simulink model "model_vec"  (R2022b)
settings: Solver=ode4  StartTime=0.0  StopTime=1.3  FixedStep=10e-6  RelTol=1e-3
InitFcn:
  | model_
values from neighbouring files (symbols this model uses):
  f = 50    [model_.m]
  i1dn = psi2n/Lm    [model_.m]
  i1qn = sqrt(Inmax^2-i1dn^2)    [model_.m]
  J = 0.4    [model_.m]
  L1 = L1sigma+Lm    (= 0.08477)    [model_.m]
  L1sigma = 2.27e-3    (= 0.00227)    [model_.m]
  L2 = L2sigma+Lm    (= 0.08477)    [model_.m]
  L2sigma = 2.27e-3    (= 0.00227)    [model_.m]
  Lm = 82.5e-3    (= 0.0825)    [model_.m]
  pp = 2    [model_.m]
  psi2n = sqrt(psi2nre^2+psi2nim^2)    [model_.m]
  R1 = 370e-3    (= 0.37)    [model_.m]
  R2 = 225e-3    (= 0.225)    [model_.m]
  R2_vec_model = 225e-3    (= 0.225)    [model_.m]
  sigma = 1-Lm^(2)/(L1*L2)    (= 0.0528396032209)    [model_.m]
  svmFrequency = 10000    [model_.m]
  Us = 400    [model_.m]
libraries: eeTransforms x16, spsMeanLib x7, slpidlib x4, simulink x2, dspsigops x2
(part 3 of 3)

== system model_vec/ASM1/i2 ==
  psi_2alpha : Inport
  psi_2beta : Inport  Port=2
  i_1_alpha_beta : Inport  Port=3
  Add2 : Sum  Inputs=+-
  Constant6 : Constant  Value=Lm
  Constant7 : Constant  Value=L2
  Divide4 : Product  Inputs=**
  Divide5 : Product  Inputs=*/
  Mux2 : Mux  Inputs=2
  i_2alpha_beta : Outport
  wires:
  i_1_alpha_beta/1 -> Divide4/1
  Divide5/1 -> i_2alpha_beta/1
  Constant7/1 -> Divide5/2
  psi_2beta/1 -> Mux2/2
  Divide4/1 -> Add2/2
  Constant6/1 -> Divide4/2
  Add2/1 -> Divide5/1
  Mux2/1 -> Add2/1
  psi_2alpha/1 -> Mux2/1

== system model_vec/ASM2/ClarkeTransform1 ==
  u_1source : Inport
  K : Inport  Port=2
  Add1 : Sum  Inputs=+++
  Add2 : Sum  Inputs=+++
  Demux4 : Demux  Outputs=3
  Demux5 : Demux  Outputs=3
  Divide2 : Product  Inputs=**
  Divide3 : Product  Inputs=**
  Gain : Gain  Gain=-1/2
  Gain1 : Gain  Gain=-1/2
  Gain2 : Gain  Gain=-sqrt(3)/2
  Gain3 : Gain  Gain=sqrt(3)/2
  Gain4 : Gain
  Gain5 : Gain  Gain=0
  Mux2 : Mux  Inputs=2
  u1_in_alpha_beta : Outport
  wires:
  Demux4/1 -> Gain4/1  "ua"
  Divide2/1 -> Mux2/1  "u_1alpha"
  [K_ClarkeTransform] -> Divide2/2
  Add1/1 -> Divide2/1
  Demux4/2 -> Gain/1  "ub"
  Divide3/1 -> Mux2/2  "u_1beta"
  Gain5/1 -> Add2/1
  Gain/1 -> Add1/2
  Demux5/1 -> Gain5/1  "ua"
  Gain3/1 -> Add2/3
  [K_ClarkeTransform] -> Divide3/2
  Gain2/1 -> Add2/2
  Gain1/1 -> Add1/3
  Demux5/2 -> Gain2/1  "ub"
  Demux5/3 -> Gain3/1  "uc"
  Add2/1 -> Divide3/1
  Gain4/1 -> Add1/1
  u_1source/1 -> Demux5/1, Demux4/1
  K/1 -> [K_ClarkeTransform]
  Mux2/1 -> u1_in_alpha_beta/1
  Demux4/3 -> Gain1/1  "uc"

== system model_vec/ASM2/Mh ==
  i_1alpha : Inport
  i_1beta : Inport  Port=2
  phi_2alpha : Inport  Port=3
  phi_2beta : Inport  Port=4
  Add : Sum  Inputs=+-
  Constant : Constant  Value=3/2
  Constant1 : Constant  Value=pp
  Constant2 : Constant  Value=Lm
  Constant3 : Constant  Value=L2
  Divide{,1,3..5} (5 alike) : Product  Inputs=**
  Divide2 : Product  Inputs=*/
  Mh : Outport
  wires:
  Constant/1 -> Divide/1
  Constant1/1 -> Divide/2
  Divide/1 -> Divide1/1
  Constant2/1 -> Divide2/1
  Constant3/1 -> Divide2/2
  Divide2/1 -> Divide1/2
  Divide1/1 -> Divide3/2
  phi_2alpha/1 -> Divide4/2
  i_1beta/1 -> Divide4/1
  Divide4/1 -> Add/1
  phi_2beta/1 -> Divide5/1
  i_1alpha/1 -> Divide5/2
  Divide5/1 -> Add/2
  Add/1 -> Divide3/1
  Divide3/1 -> Mh/1

== system model_vec/ASM2/Mh Static ==
  Slip : Inport
  Add3 : Sum
  Add4 : Sum
  Add6 : Sum
  Constant10 : Constant  Value=230^(2)
  Constant11 : Constant  Value=pp
  Constant14 : Constant  Value=2*pi*f
  Constant15 : Constant  Value=R1
  Constant16 : Constant  Value=R2
  Constant21 : Constant  Value=2*pi*f
  Constant22 : Constant  Value=L1sigma
  Constant23 : Constant  Value=L2sigma
  Constant8 : Constant  Value=3
  Constant9 : Constant  Value=R2
  Divide10 : Product  Inputs=/*
  Divide11 : Product  Inputs=*/
  Divide15 : Product  Inputs=**
  Divide6 : Product  Inputs=****
  Divide7 : Product  Inputs=*/
  Divide8 : Product  Inputs=**
  Math Function : Math  Operator=square
  Math Function2 : Math  Operator=square
  Reprezentace s s*omega1*L2sigma : Subsystem
  Mh Static : Outport
  wires:
  Slip/1 -> Divide8/2, Divide11/2
  Constant11/1 -> Divide6/4
  Constant10/1 -> Divide6/3
  Add4/1 -> Math Function/1
  Constant16/1 -> Divide11/1
  Constant9/1 -> Divide6/2
  Constant23/1 -> Add6/2
  Constant15/1 -> Add4/1
  Divide15/1 -> Math Function2/1
  Divide8/1 -> Divide7/2
  Constant14/1 -> Divide8/1
  Math Function/1 -> Add3/1
  Divide7/1 -> Divide10/2
  Divide10/1 -> Mh Static/1
  Divide11/1 -> Add4/2
  Constant22/1 -> Add6/1
  Add6/1 -> Divide15/1
  Constant8/1 -> Divide6/1
  Constant21/1 -> Divide15/2
  Add3/1 -> Divide10/1
  Divide6/1 -> Divide7/1
  Math Function2/1 -> Add3/2

== system model_vec/ASM2/Slip ==
  omega : Inport
  Add2 : Sum  Inputs=+-
  Constant12 : Constant  Value=2*pi*f
  Constant13 : Constant  Value=2*pi*f
  Divide9 : Product  Inputs=*/
  Slip : Outport
  wires:
  omega/1 -> Add2/2  "Omega"
  Divide9/1 -> Slip/1
  Constant12/1 -> Add2/1
  Add2/1 -> Divide9/1
  Constant13/1 -> Divide9/2

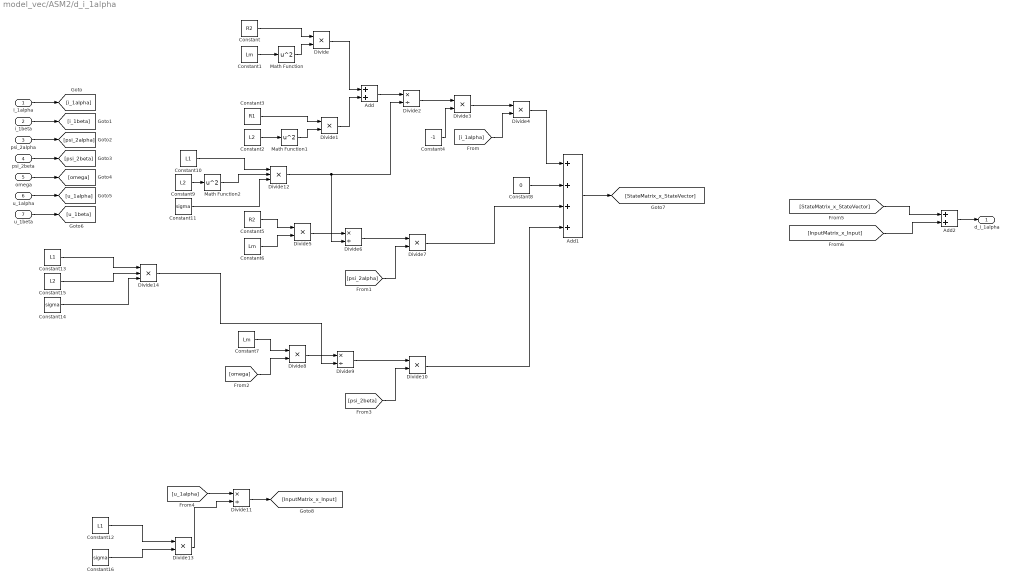
== system model_vec/ASM2/d_i_1alpha ==
  i_1alpha : Inport
  i_1beta : Inport  Port=2
  psi_2alpha : Inport  Port=3
  psi_2beta : Inport  Port=4
  omega : Inport  Port=5
  u_1alpha : Inport  Port=6
  u_1beta : Inport  Port=7
  Add : Sum
  Add1 : Sum  Inputs=++++
  Add2 : Sum
  Constant : Constant  Value=R2
  Constant1 : Constant  Value=Lm
  Constant10 : Constant  Value=L1
  Constant11 : Constant  Value=sigma
  Constant12 : Constant  Value=L1
  Constant13 : Constant  Value=L1
  Constant14 : Constant  Value=sigma
  Constant15 : Constant  Value=L2
  Constant16 : Constant  Value=sigma
  Constant2 : Constant  Value=L2
  Constant3 : Constant  Value=R1
  Constant4 : Constant  Value=-1
  Constant5 : Constant  Value=R2
  Constant6 : Constant  Value=Lm
  Constant7 : Constant  Value=Lm
  Constant8 : Constant  Value=0
  Constant9 : Constant  Value=L2
  Divide{,1,3..5,7..8,10,13} (9 alike) : Product  Inputs=**
  Divide{2,6,9,11} (4 alike) : Product  Inputs=*/
  Divide12 : Product  Inputs=***
  Divide14 : Product  Inputs=***
  Math Function : Math  Operator=square
  Math Function1 : Math  Operator=square
  Math Function2 : Math  Operator=square
  d_i_1alpha : Outport
  wires:
  Constant1/1 -> Math Function/1
  Constant/1 -> Divide/1
  Math Function/1 -> Divide/2
  Divide/1 -> Add/1
  Constant2/1 -> Math Function1/1
  Constant3/1 -> Divide1/1
  Math Function1/1 -> Divide1/2
  Divide1/1 -> Add/2
  Add/1 -> Divide2/1
  Constant4/1 -> Divide3/2
  Divide2/1 -> Divide3/1
  Divide3/1 -> Divide4/1
  i_1alpha/1 -> [i_1alpha]
  i_1beta/1 -> [i_1beta]
  psi_2alpha/1 -> [psi_2alpha]
  psi_2beta/1 -> [psi_2beta]
  omega/1 -> [omega]
  [i_1alpha] -> Divide4/2
  Divide4/1 -> Add1/1
  Constant5/1 -> Divide5/1
  Constant6/1 -> Divide5/2
  Divide5/1 -> Divide6/1
  Divide6/1 -> Divide7/1
  [psi_2alpha] -> Divide7/2
  Divide7/1 -> Add1/3
  Constant7/1 -> Divide8/1
  [omega] -> Divide8/2
  Divide8/1 -> Divide9/1
  Divide9/1 -> Divide10/1
  [psi_2beta] -> Divide10/2
  Divide10/1 -> Add1/4
  Constant8/1 -> Add1/2
  u_1alpha/1 -> [u_1alpha]
  u_1beta/1 -> [u_1beta]
  Add1/1 -> [StateMatrix_x_StateVector]
  [u_1alpha] -> Divide11/1
  Divide11/1 -> [InputMatrix_x_Input]
  [StateMatrix_x_StateVector] -> Add2/1
  [InputMatrix_x_Input] -> Add2/2
  Add2/1 -> d_i_1alpha/1
  Constant9/1 -> Math Function2/1
  Constant10/1 -> Divide12/1
  Math Function2/1 -> Divide12/2
  Constant11/1 -> Divide12/3
  Divide12/1 -> Divide6/2, Divide2/2
  Constant14/1 -> Divide14/3
  Constant13/1 -> Divide14/1
  Constant15/1 -> Divide14/2
  Constant12/1 -> Divide13/1
  Constant16/1 -> Divide13/2
  Divide13/1 -> Divide11/2
  Divide14/1 -> Divide9/2

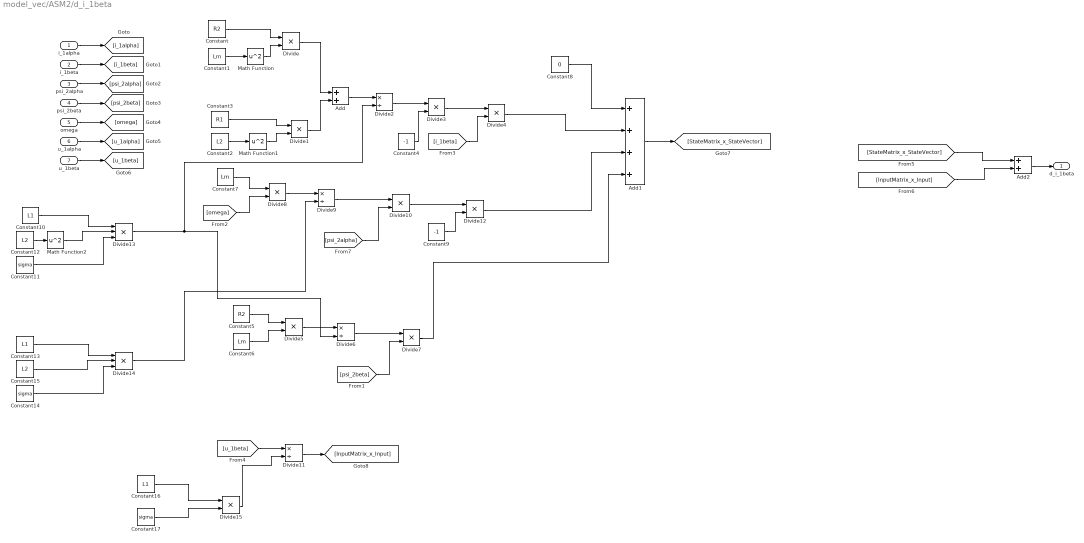
== system model_vec/ASM2/d_i_1beta ==
  i_1alpha : Inport
  i_1beta : Inport  Port=2
  psi_2alpha : Inport  Port=3
  psi_2beta : Inport  Port=4
  omega : Inport  Port=5
  u_1alpha : Inport  Port=6
  u_1beta : Inport  Port=7
  Add : Sum
  Add1 : Sum  Inputs=++++
  Add2 : Sum
  Constant : Constant  Value=R2
  Constant1 : Constant  Value=Lm
  Constant10 : Constant  Value=L1
  Constant11 : Constant  Value=sigma
  Constant12 : Constant  Value=L2
  Constant13 : Constant  Value=L1
  Constant14 : Constant  Value=sigma
  Constant15 : Constant  Value=L2
  Constant16 : Constant  Value=L1
  Constant17 : Constant  Value=sigma
  Constant2 : Constant  Value=L2
  Constant3 : Constant  Value=R1
  Constant4 : Constant  Value=-1
  Constant5 : Constant  Value=R2
  Constant6 : Constant  Value=Lm
  Constant7 : Constant  Value=Lm
  Constant8 : Constant  Value=0
  Constant9 : Constant  Value=-1
  Divide{,1,3..5,7..8,10,12,15} (10 alike) : Product  Inputs=**
  Divide{2,6,9,11} (4 alike) : Product  Inputs=*/
  Divide13 : Product  Inputs=***
  Divide14 : Product  Inputs=***
  Math Function : Math  Operator=square
  Math Function1 : Math  Operator=square
  Math Function2 : Math  Operator=square
  d_i_1beta : Outport
  wires:
  Add2/1 -> d_i_1beta/1
  [InputMatrix_x_Input] -> Add2/2
  [StateMatrix_x_StateVector] -> Add2/1
  Divide11/1 -> [InputMatrix_x_Input]
  [u_1beta] -> Divide11/1
  Add1/1 -> [StateMatrix_x_StateVector]
  u_1beta/1 -> [u_1beta]
  u_1alpha/1 -> [u_1alpha]
  Constant8/1 -> Add1/1
  Divide10/1 -> Divide12/1
  [psi_2alpha] -> Divide10/2
  Divide9/1 -> Divide10/1
  Divide8/1 -> Divide9/1
  [omega] -> Divide8/2
  Constant7/1 -> Divide8/1
  Divide7/1 -> Add1/4
  [psi_2beta] -> Divide7/2
  Divide6/1 -> Divide7/1
  Divide5/1 -> Divide6/1
  Constant6/1 -> Divide5/2
  Constant5/1 -> Divide5/1
  Divide4/1 -> Add1/2
  [i_1beta] -> Divide4/2
  omega/1 -> [omega]
  psi_2beta/1 -> [psi_2beta]
  psi_2alpha/1 -> [psi_2alpha]
  i_1beta/1 -> [i_1beta]
  i_1alpha/1 -> [i_1alpha]
  Divide3/1 -> Divide4/1
  Divide2/1 -> Divide3/1
  Constant4/1 -> Divide3/2
  Add/1 -> Divide2/1
  Divide1/1 -> Add/2
  Math Function1/1 -> Divide1/2
  Constant3/1 -> Divide1/1
  Constant2/1 -> Math Function1/1
  Divide/1 -> Add/1
  Math Function/1 -> Divide/2
  Constant/1 -> Divide/1
  Constant1/1 -> Math Function/1
  Constant9/1 -> Divide12/2
  Divide12/1 -> Add1/3
  Constant10/1 -> Divide13/1
  Constant11/1 -> Divide13/3
  Math Function2/1 -> Divide13/2
  Divide13/1 -> Divide6/2, Divide2/2
  Constant12/1 -> Math Function2/1
  Divide14/1 -> Divide9/2
  Constant14/1 -> Divide14/3
  Constant15/1 -> Divide14/2
  Constant13/1 -> Divide14/1
  Constant16/1 -> Divide15/1
  Divide15/1 -> Divide11/2
  Constant17/1 -> Divide15/2

== system model_vec/ASM2/d_psi_2alpha ==
  note: je to jen pro úplnost
  i_1alpha : Inport
  i_1beta : Inport  Port=2
  psi_2alpha : Inport  Port=3
  psi_2beta : Inport  Port=4
  omega : Inport  Port=5
  u_1alpha : Inport  Port=6
  u_1beta : Inport  Port=7
  Add1 : Sum  Inputs=++++
  Add2 : Sum
  Constant : Constant  Value=0
  Constant1 : Constant  Value=-1
  Constant2 : Constant  Value=-1
  Constant3 : Constant  Value=R2
  Constant4 : Constant  Value=L2
  Constant5 : Constant  Value=Lm
  Constant6 : Constant  Value=R2
  Constant7 : Constant  Value=L2
  Constant8 : Constant  Value=0
  Divide{,1,3..5,7} (6 alike) : Product  Inputs=**
  Divide2 : Product  Inputs=*/
  Divide6 : Product  Inputs=*/
  d_psi_2alpha : Outport
  wires:
  i_1alpha/1 -> [i_1alpha]
  i_1beta/1 -> [i_1beta]
  psi_2alpha/1 -> [psi_2alpha]
  psi_2beta/1 -> [psi_2beta]
  omega/1 -> [omega]
  Constant8/1 -> Add1/2
  u_1alpha/1 -> [u_1alpha]
  u_1beta/1 -> [u_1beta]
  Add1/1 -> [StateMatrix_x_StateVector]
  Constant/1 -> [InputMatrix_x_Input]
  [StateMatrix_x_StateVector] -> Add2/1
  [InputMatrix_x_Input] -> Add2/2
  Add2/1 -> d_psi_2alpha/1
  [omega] -> Divide/1
  Constant1/1 -> Divide/2
  Divide/1 -> Divide1/1
  [psi_2beta] -> Divide1/2
  Divide1/1 -> Add1/4
  Constant2/1 -> Divide3/2
  Divide2/1 -> Divide3/1
  Constant3/1 -> Divide2/1
  Constant4/1 -> Divide2/2
  Divide3/1 -> Divide4/1
  [psi_2alpha] -> Divide4/2
  Divide4/1 -> Add1/3
  Divide5/1 -> Divide6/1
  Constant5/1 -> Divide5/1
  Constant6/1 -> Divide5/2
  Constant7/1 -> Divide6/2
  Divide6/1 -> Divide7/1
  [i_1alpha] -> Divide7/2
  Divide7/1 -> Add1/1

== system model_vec/ASM2/d_psi_2beta ==
  i_1alpha : Inport
  i_1beta : Inport  Port=2
  psi_2alpha : Inport  Port=3
  psi_2beta : Inport  Port=4
  omega : Inport  Port=5
  u_1alpha : Inport  Port=6
  u_1beta : Inport  Port=7
  Add1 : Sum  Inputs=++++
  Add2 : Sum
  Constant : Constant  Value=0
  Constant2 : Constant  Value=-1
  Constant3 : Constant  Value=R2
  Constant4 : Constant  Value=L2
  Constant5 : Constant  Value=Lm
  Constant6 : Constant  Value=R2
  Constant7 : Constant  Value=L2
  Constant8 : Constant  Value=0
  Divide{1,3..5,7} (5 alike) : Product  Inputs=**
  Divide2 : Product  Inputs=*/
  Divide6 : Product  Inputs=*/
  d_psi_2beta : Outport
  wires:
  Divide7/1 -> Add1/2
  [i_1beta] -> Divide7/2
  Divide6/1 -> Divide7/1
  Constant7/1 -> Divide6/2
  Constant6/1 -> Divide5/2
  Constant5/1 -> Divide5/1
  Divide5/1 -> Divide6/1
  Divide4/1 -> Add1/4
  [psi_2beta] -> Divide4/2
  Divide3/1 -> Divide4/1
  Constant4/1 -> Divide2/2
  Constant3/1 -> Divide2/1
  Divide2/1 -> Divide3/1
  Constant2/1 -> Divide3/2
  Divide1/1 -> Add1/3
  [psi_2alpha] -> Divide1/2
  Add2/1 -> d_psi_2beta/1
  [InputMatrix_x_Input] -> Add2/2
  [StateMatrix_x_StateVector] -> Add2/1
  Constant/1 -> [InputMatrix_x_Input]
  Add1/1 -> [StateMatrix_x_StateVector]
  u_1beta/1 -> [u_1beta]
  u_1alpha/1 -> [u_1alpha]
  Constant8/1 -> Add1/1
  omega/1 -> [omega]
  psi_2beta/1 -> [psi_2beta]
  psi_2alpha/1 -> [psi_2alpha]
  i_1beta/1 -> [i_1beta]
  i_1alpha/1 -> [i_1alpha]
  [omega] -> Divide1/1

== system model_vec/ASM2/i2 ==
  psi_2alpha : Inport
  psi_2beta : Inport  Port=2
  i_1_alpha_beta : Inport  Port=3
  Add2 : Sum  Inputs=+-
  Constant6 : Constant  Value=Lm
  Constant7 : Constant  Value=L2
  Divide4 : Product  Inputs=**
  Divide5 : Product  Inputs=*/
  Mux2 : Mux  Inputs=2
  i_2alpha_beta : Outport
  wires:
  psi_2alpha/1 -> Mux2/1
  Mux2/1 -> Add2/1
  Add2/1 -> Divide5/1
  Constant6/1 -> Divide4/2
  Divide4/1 -> Add2/2
  psi_2beta/1 -> Mux2/2
  Constant7/1 -> Divide5/2
  Divide5/1 -> i_2alpha_beta/1
  i_1_alpha_beta/1 -> Divide4/1

== system model_vec/Goniometric Space Vector Modulation Invertor/Comparation of Signal with Triangle Wave ==
  sine1 : Inport
  sine2 : Inport  Port=2
  sine3 : Inport  Port=3
  Logical Operator : Logic  Operator=NOT  AllPortsSameDT=off  OutDataTypeStr=boolean
  Logical Operator1 : Logic  Operator=NOT  AllPortsSameDT=off  OutDataTypeStr=boolean
  Logical Operator2 : Logic  Operator=NOT  AllPortsSameDT=off  OutDataTypeStr=boolean
  Mux : Mux  Inputs=2
  Relational Operator : RelationalOperator  Operator=<=  OutDataTypeStr=boolean  RndMeth=Simplest  InputSameDT=off
  Relational Operator1 : RelationalOperator  Operator=<=  OutDataTypeStr=boolean  RndMeth=Simplest  InputSameDT=off
  Relational Operator2 : RelationalOperator  Operator=<=  OutDataTypeStr=boolean  RndMeth=Simplest  InputSameDT=off
  Repeating Sequence : simulink/Sources/Repeating Sequence  rep_seq_t=TriangleTime10kHz  rep_seq_y=TriangleData
  Scope : Scope
  Sw1 : Outport
  Sw2 : Outport  Port=2
  Sw3 : Outport  Port=3
  Sw4 : Outport  Port=4
  Sw5 : Outport  Port=5
  Sw6 : Outport  Port=6
  wires:
  sine1/1 -> Mux/2, Relational Operator/1
  Relational Operator/1 -> Logical Operator/1, Sw1/1
  Repeating Sequence/1 -> Mux/1, Relational Operator/2, Relational Operator1/2, Relational Operator2/2
  Logical Operator/1 -> Sw4/1
  sine2/1 -> Relational Operator1/1
  sine3/1 -> Relational Operator2/1
  Relational Operator1/1 -> Sw3/1, Logical Operator1/1
  Logical Operator1/1 -> Sw6/1
  Relational Operator2/1 -> Sw5/1, Logical Operator2/1
  Logical Operator2/1 -> Sw2/1
  Mux/1 -> Scope/1

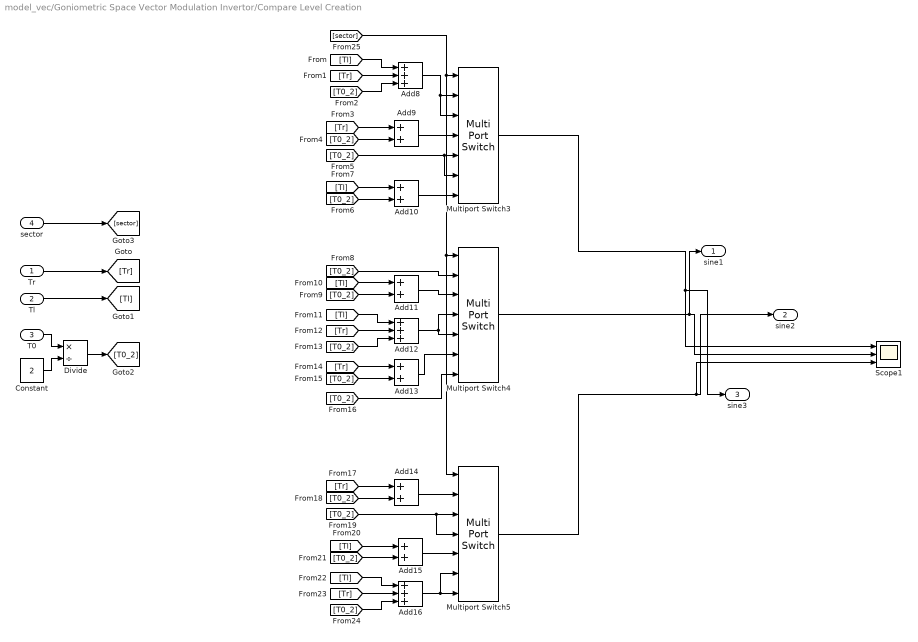
== system model_vec/Goniometric Space Vector Modulation Invertor/Compare Level Creation ==
  Tr : Inport
  Tl : Inport  Port=2
  T0 : Inport  Port=3
  sector : Inport  Port=4
  Add{9..11,13..15} (6 alike) : Sum
  Add12 : Sum  Inputs=+++
  Add16 : Sum  Inputs=+++
  Add8 : Sum  Inputs=+++
  Constant : Constant  Value=2
  Divide : Product  Inputs=*/
  Multiport Switch3 : MultiPortSwitch  Inputs=6  DiagnosticForDefault=None  SaturateOnIntegerOverflow=off  InputSameDT=off
  Multiport Switch4 : MultiPortSwitch  Inputs=6  DiagnosticForDefault=None  SaturateOnIntegerOverflow=off  InputSameDT=off
  Multiport Switch5 : MultiPortSwitch  Inputs=6  DiagnosticForDefault=None  SaturateOnIntegerOverflow=off  InputSameDT=off
  Scope1 : Scope  NumInputPorts=3
  sine1 : Outport
  sine2 : Outport  Port=2
  sine3 : Outport  Port=3
  wires:
  sector/1 -> [sector]
  T0/1 -> Divide/1
  Constant/1 -> Divide/2
  Tr/1 -> [Tr]
  Tl/1 -> [Tl]
  Divide/1 -> [T0_2]
  [Tl] -> Add8/1
  [Tr] -> Add8/2
  [T0_2] -> Add8/3
  Add8/1 -> Multiport Switch3/3, Multiport Switch3/2
  [Tr] -> Add9/1
  [T0_2] -> Add9/2
  Add9/1 -> Multiport Switch3/4
  [T0_2] -> Multiport Switch3/6, Multiport Switch3/5
  [T0_2] -> Add10/2
  [Tl] -> Add10/1
  Add10/1 -> Multiport Switch3/7
  [T0_2] -> Multiport Switch4/2
  Add11/1 -> Multiport Switch4/3
  [T0_2] -> Add11/2
  [T0_2] -> Add12/3
  [Tr] -> Add12/2
  [Tl] -> Add12/1
  Add12/1 -> Multiport Switch4/5, Multiport Switch4/4
  [Tl] -> Add11/1
  [T0_2] -> Add13/2
  [Tr] -> Add13/1
  Add13/1 -> Multiport Switch4/6
  [T0_2] -> Multiport Switch4/7
  [Tr] -> Add14/1
  [T0_2] -> Add14/2
  Add14/1 -> Multiport Switch5/2
  [T0_2] -> Multiport Switch5/4, Multiport Switch5/3
  [T0_2] -> Add15/2
  [Tl] -> Add15/1
  Add15/1 -> Multiport Switch5/5
  [Tl] -> Add16/1
  [Tr] -> Add16/2
  [T0_2] -> Add16/3
  Add16/1 -> Multiport Switch5/7, Multiport Switch5/6
  [sector] -> Multiport Switch5/1, Multiport Switch4/1, Multiport Switch3/1
  Multiport Switch3/1 -> sine3/1, Scope1/1
  Multiport Switch4/1 -> Scope1/2, sine1/1
  Multiport Switch5/1 -> sine2/1, Scope1/3

== system model_vec/Goniometric Space Vector Modulation Invertor/Output Voltage of Inverter Reconstruction ==
  note: reconstruction of Ua voltage
  note: reconstruction of Ub voltage
  note: reconstruction of Uc voltage
  note: sources
  Sa : Inport
  Sb : Inport  Port=2
  Sc : Inport  Port=3
  uDC : Inport  Port=4
  Add : Sum  Inputs=+++
  Add1 : Sum  Inputs=+++
  Add2 : Sum  Inputs=+++
  Constant : Constant  Value=2
  Constant{1..2,5..6,8} (5 alike) : Constant  Value=-1
  Constant3 : Constant  Value=1/3
  Constant4 : Constant  Value=2
  Constant7 : Constant  Value=2
  Divide{,1..12} (13 alike) : Product  Inputs=**
  u1 : Outport
  u2 : Outport  Port=2
  u3 : Outport  Port=3
  wires:
  Constant/1 -> Divide/2
  Constant1/1 -> Divide1/1, Divide2/2
  Divide/1 -> Add/1
  Divide1/1 -> Add/2
  Divide2/1 -> Add/3
  Constant2/1 -> Divide3/1
  Add/1 -> Divide4/1
  uDC/1 -> Divide5/1
  Constant3/1 -> Divide5/2
  Divide4/1 -> u1/1
  Sa/1 -> [Sa]
  Sb/1 -> [Sb]
  Sc/1 -> [Sc]
  Divide5/1 -> [uDC]
  [Sa] -> Divide/1
  [Sb] -> Divide1/2
  [Sc] -> Divide2/1
  [uDC] -> Divide4/2
  [Sa] -> Divide3/2
  Constant4/1 -> Divide6/2
  [Sb] -> Divide6/1
  [Sc] -> Divide7/2
  Constant5/1 -> Divide7/1
  Divide3/1 -> Add1/1
  Divide6/1 -> Add1/2
  Divide7/1 -> Add1/3
  Add1/1 -> Divide8/1
  [uDC] -> Divide8/2
  Divide8/1 -> u2/1
  [uDC] -> Divide12/2
  Add2/1 -> Divide12/1
  Divide9/1 -> Add2/1
  Constant8/1 -> Divide11/1
  [Sb] -> Divide11/2
  [Sc] -> Divide10/1
  Constant7/1 -> Divide10/2
  [Sa] -> Divide9/2
  Constant6/1 -> Divide9/1
  Divide11/1 -> Add2/2
  Divide10/1 -> Add2/3
  Divide12/1 -> u3/1

== system model_vec/I-n model/Module of Vector1 ==
  In1 : Inport
  In2 : Inport  Port=2
  Add2 : Sum
  Math Function : Math  Operator=square
  Math Function1 : Math  Operator=square
  Sqrt : Sqrt
  Psi : Outport
  wires:
  Add2/1 -> Sqrt/1
  In2/1 -> Math Function1/1
  Math Function1/1 -> Add2/2
  Math Function/1 -> Add2/1
  Sqrt/1 -> Psi/1
  In1/1 -> Math Function/1

== system model_vec/Min-Max Method Space Vector Modulation Invertor/Comparation of Signal with Triangle Wave ==
  sine1 : Inport
  sine2 : Inport  Port=2
  sine3 : Inport  Port=3
  Logical Operator : Logic  Operator=NOT  AllPortsSameDT=off  OutDataTypeStr=boolean
  Logical Operator1 : Logic  Operator=NOT  AllPortsSameDT=off  OutDataTypeStr=boolean
  Logical Operator2 : Logic  Operator=NOT  AllPortsSameDT=off  OutDataTypeStr=boolean
  Mux : Mux  Inputs=2
  Relational Operator : RelationalOperator  OutDataTypeStr=boolean  RndMeth=Simplest  InputSameDT=off
  Relational Operator1 : RelationalOperator  OutDataTypeStr=boolean  RndMeth=Simplest  InputSameDT=off
  Relational Operator2 : RelationalOperator  OutDataTypeStr=boolean  RndMeth=Simplest  InputSameDT=off
  Repeating Sequence : simulink/Sources/Repeating Sequence  rep_seq_t=TriangleTime10kHz  rep_seq_y=[-1,1,-1]
  Scope : Scope
  Sw1 : Outport
  Sw2 : Outport  Port=2
  Sw3 : Outport  Port=3
  Sw4 : Outport  Port=4
  Sw5 : Outport  Port=5
  Sw6 : Outport  Port=6
  wires:
  sine1/1 -> Mux/2, Relational Operator/1
  Relational Operator/1 -> Logical Operator/1, Sw1/1
  Repeating Sequence/1 -> Mux/1, Relational Operator/2, Relational Operator1/2, Relational Operator2/2
  Logical Operator/1 -> Sw4/1
  sine2/1 -> Relational Operator1/1
  sine3/1 -> Relational Operator2/1
  Relational Operator1/1 -> Sw3/1, Logical Operator1/1
  Logical Operator1/1 -> Sw6/1
  Relational Operator2/1 -> Sw5/1, Logical Operator2/1
  Logical Operator2/1 -> Sw2/1
  Mux/1 -> Scope/1

== system model_vec/Min-Max Method Space Vector Modulation Invertor/Output Voltage of Inverter Reconstruction ==
  note: reconstruction of Ua voltage
  note: reconstruction of Ub voltage
  note: reconstruction of Uc voltage
  note: sources
  Sa : Inport
  Sb : Inport  Port=2
  Sc : Inport  Port=3
  uDC : Inport  Port=4
  Add : Sum  Inputs=+++
  Add1 : Sum  Inputs=+++
  Add2 : Sum  Inputs=+++
  Constant : Constant  Value=2
  Constant{1..2,5..6,8} (5 alike) : Constant  Value=-1
  Constant3 : Constant  Value=1/3
  Constant4 : Constant  Value=2
  Constant7 : Constant  Value=2
  Divide{,1..12} (13 alike) : Product  Inputs=**
  Gain3 : Gain  Gain=-1
  u1 : Outport
  u2 : Outport  Port=2
  u3 : Outport  Port=3
  wires:
  Constant/1 -> Divide/2
  Constant1/1 -> Divide1/1, Divide2/2
  Divide/1 -> Add/1
  Divide1/1 -> Add/2
  Divide2/1 -> Add/3
  Constant2/1 -> Divide3/1
  Add/1 -> Divide4/1
  uDC/1 -> Divide5/1
  Constant3/1 -> Divide5/2
  Sa/1 -> [Sa]
  Sb/1 -> [Sb]
  Sc/1 -> [Sc]
  Divide5/1 -> [uDC]
  [Sa] -> Divide/1
  [Sb] -> Divide1/2
  [Sc] -> Divide2/1
  [uDC] -> Divide4/2
  [Sa] -> Divide3/2
  Constant4/1 -> Divide6/2
  [Sb] -> Divide6/1
  [Sc] -> Divide7/2
  Constant5/1 -> Divide7/1
  Divide3/1 -> Add1/1
  Divide6/1 -> Add1/2
  Divide7/1 -> Add1/3
  Add1/1 -> Divide8/1
  [uDC] -> Divide8/2
  [uDC] -> Divide12/2
  Add2/1 -> Divide12/1
  Divide9/1 -> Add2/1
  Constant8/1 -> Divide11/1
  [Sb] -> Divide11/2
  [Sc] -> Divide10/1
  Constant7/1 -> Divide10/2
  [Sa] -> Divide9/2
  Constant6/1 -> Divide9/1
  Divide11/1 -> Add2/2
  Divide10/1 -> Add2/3
  Divide8/1 -> u2/1
  Divide12/1 -> u3/1
  Divide4/1 -> u1/1

== system model_vec/ASM/Mh Static/Reprezentace s s*omega1*L2sigma ==
  Slip : Inport
  Add5 : Sum
  Constant17 : Constant  Value=2*pi*f
  Constant18 : Constant  Value=L1sigma
  Constant19 : Constant  Value=L2sigma
  Constant20 : Constant  Value=2*pi*f
  Divide12 : Product  Inputs=**
  Divide13 : Product  Inputs=**
  Divide14 : Product  Inputs=**
  Out1 : Outport
  wires:
  Divide13/1 -> Add5/2
  Divide14/1 -> Divide13/1
  Add5/1 -> Out1/1
  Constant18/1 -> Divide12/1
  Slip/1 -> Divide14/1
  Constant17/1 -> Divide12/2
  Divide12/1 -> Add5/1
  Constant20/1 -> Divide14/2
  Constant19/1 -> Divide13/2

== system model_vec/ASM1/Mh Static/Reprezentace s s*omega1*L2sigma ==
  Slip : Inport
  Add5 : Sum
  Constant17 : Constant  Value=2*pi*f
  Constant18 : Constant  Value=L1sigma
  Constant19 : Constant  Value=L2sigma
  Constant20 : Constant  Value=2*pi*f
  Divide12 : Product  Inputs=**
  Divide13 : Product  Inputs=**
  Divide14 : Product  Inputs=**
  Out1 : Outport
  wires:
  Constant19/1 -> Divide13/2
  Constant20/1 -> Divide14/2
  Divide12/1 -> Add5/1
  Constant17/1 -> Divide12/2
  Slip/1 -> Divide14/1
  Constant18/1 -> Divide12/1
  Add5/1 -> Out1/1
  Divide14/1 -> Divide13/1
  Divide13/1 -> Add5/2

== system model_vec/ASM2/Mh Static/Reprezentace s s*omega1*L2sigma ==
  Slip : Inport
  Add5 : Sum
  Constant17 : Constant  Value=2*pi*f
  Constant18 : Constant  Value=L1sigma
  Constant19 : Constant  Value=L2sigma
  Constant20 : Constant  Value=2*pi*f
  Divide12 : Product  Inputs=**
  Divide13 : Product  Inputs=**
  Divide14 : Product  Inputs=**
  Out1 : Outport
  wires:
  Divide13/1 -> Add5/2
  Divide14/1 -> Divide13/1
  Add5/1 -> Out1/1
  Constant18/1 -> Divide12/1
  Slip/1 -> Divide14/1
  Constant17/1 -> Divide12/2
  Divide12/1 -> Add5/1
  Constant20/1 -> Divide14/2
  Constant19/1 -> Divide13/2

== matlab function model_vec/Min-Max Method Space Vector Modulation Invertor/From Us to UdAV0 and uDCmax ==
  data: Us input; uDCmax output; uDC output
function [uDCmax, uDC] = fcn(Us)
% uDC=UdAV0

uDCmax = (3*sqrt(2))/(pi*sqrt(3))*Us;
uDC = (3*sqrt(2))/(pi)*Us;

== matlab function model_vec/Goniometric Space Vector Modulation Invertor/From Us to UdAV0 and uDCmax ==
  data: Us input; uDCmax output; uDC output
function [uDCmax, uDC] = fcn(Us)
% uDC=UdAV0

uDCmax = (3*sqrt(2))/(pi*sqrt(3))*Us;
uDC = (3*sqrt(2))/(pi)*Us;

== matlab function model_vec/Goniometric Space Vector Modulation Invertor/Converting Angle To Sector ==
  data: angle input; sector output
function sector = fcn(angle)

if (angle>0) && (angle <= pi/3)
    sector = 1;
elseif (angle>pi/3) && (angle <= 2*pi/3)
    sector = 2;
elseif (angle>2*pi/3) && (angle <= pi)
    sector = 3;
elseif (angle>-pi) && (angle <= -2*pi/3)
    sector = 4;
elseif (angle>-2*pi/3) && (angle <= -pi/3)
    sector = 5;
elseif (angle>-pi/3) && (angle <= 0)
    sector = 6;
else
    sector=1;
end

== matlab function model_vec/Goniometric Space Vector Modulation Invertor/Switching Time Calculation ==
  data: angle input; Tr output; Tl output; T0 output; Tpwm input; uDC input; uWantedSize input; sector input
function [Tr,Tl,T0] = fcn(angle,Tpwm,uDC,uWantedSize,sector)

Tr=(((sqrt(3)*Tpwm*uWantedSize)/uDC)*(sin(pi/3 - angle + ((sector-1)/3)*pi)))/Tpwm; %T1
Tl=(((sqrt(3)*Tpwm*uWantedSize)/uDC)*sin(angle-((sector-1)/3)*pi))/Tpwm; %T2
T0=(Tpwm/Tpwm-Tl-Tr); %T0
end
